simulink model "Feedforward_completo"  (R2021b)
settings: Solver=VariableStepAuto  StartTime=0.0  StopTime=10.0  RelTol=1e-3
PreLoadFcn:
  | Fs = 44100;
  | f_tono = 500;
  | L = 32;
InitFcn:
  | Fs = 44100;
  | f_tono = 500;
  | L = 32;
undefined symbols (not defined in the file or in its folder): SzEstimado
settings Model: Creator=Vale Oieni  LastModifiedBy=ValeOieni

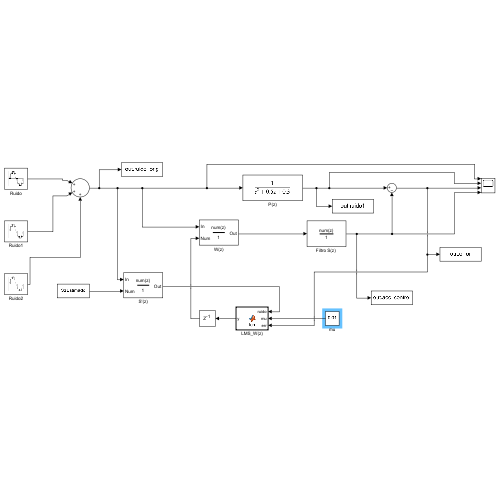
[thumbnail: Simulink's stored preview of the top-level diagram]
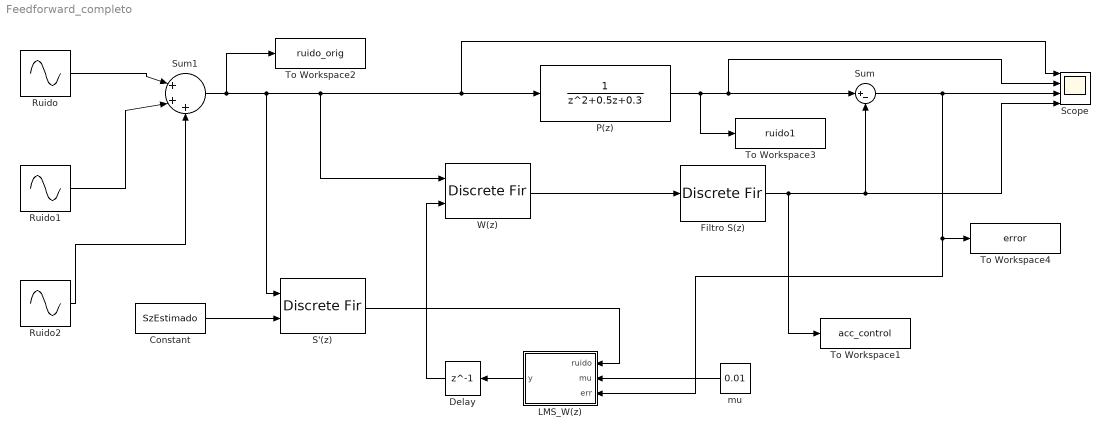
== system Feedforward_completo ==
  Constant : Constant  Value=SzEstimado  SampleTime=1/Fs
  Delay : Delay  DelayLength=1  InitialCondition=0  SampleTime=1/Fs
  "Filtro S(z) " : DiscreteFir  Coefficients=[0 0 -.5 .5 -.3 .2 -.1 .5 -.5]  InputProcessing=Columns as channels (frame based)  SampleTime=1/Fs
  LMS_W(z) : MATLAB Function  TreatAsAtomicUnit=on
  P(z) : DiscreteTransferFcn  Denominator="[1 0.5  0.3]"
  Ruido : Sin  Frequency=f_tono*(2*pi)  SampleTime=1/Fs
  Ruido1 : Sin  Frequency=2*f_tono*(2*pi)  SampleTime=1/Fs
  Ruido2 : Sin  Amplitude=2  Frequency=0.3*f_tono*(2*pi)  SampleTime=1/Fs
  S'(z) : DiscreteFir  CoefSource=Input port  InputProcessing=Columns as channels (frame based)  SampleTime=1/Fs
      settings: InputPortMap=u0,u1
  Scope : Scope  NumInputPorts=4
  Sum : Sum  Inputs=|+-
  Sum1 : Sum  Inputs=|+++
  To Workspace1 : ToWorkspace  VariableName=acc_control  SampleTime=-1
      settings: Save2DSignal=2-D array (concatenate along first dimension)
  To Workspace2 : ToWorkspace  VariableName=ruido_orig  SampleTime=-1
      settings: Save2DSignal=2-D array (concatenate along first dimension)
  To Workspace3 : ToWorkspace  VariableName=ruido1  SampleTime=-1
      settings: Save2DSignal=2-D array (concatenate along first dimension)
  To Workspace4 : ToWorkspace  VariableName=error  SampleTime=-1
      settings: Save2DSignal=2-D array (concatenate along first dimension)
  W(z) : DiscreteFir  CoefSource=Input port  SampleTime=1/Fs
      settings: InputPortMap=u0,u1
  mu : Constant  Value=0.01  SampleTime=1/Fs
  wires:
  P(z)/1 -> To Workspace3/1, Scope/2, Sum/1
  Sum/1 -> Scope/3, To Workspace4/1, LMS_W(z)/3(err)
  "Filtro S(z) "/1 -> To Workspace1/1, Scope/4, Sum/2
  Ruido/1 -> Sum1/1
  Ruido1/1 -> Sum1/2
  Ruido2/1 -> Sum1/3
  Sum1/1 -> To Workspace2/1, S'(z)/1, Scope/1, P(z)/1, W(z)/1
  W(z)/1 -> "Filtro S(z) "/1
  Constant/1 -> S'(z)/2
  S'(z)/1 -> LMS_W(z)/1(ruido)
  mu/1 -> LMS_W(z)/2(mu)
  LMS_W(z)/1(y) -> Delay/1
  Delay/1 -> W(z)/2

== matlab function Feedforward_completo/LMS_W(z) ==
  data: ruido input; mu input; y output; err input
function y = fcn(ruido, mu, err)
    L = 32;
    %Pesos w_n
    persistent w_n
    if isempty(w_n)
        w_n = zeros(1, L); % inicializa w en cero, largo L
    end
    %Vector de ruido
    persistent x
    if isempty(x)
        x = zeros(1, L); % inicializa x en cero, largo L
    end
    %Vaciado de x
    x(2:L) = x(1:L-1);
    x(1) = ruido;
    %Actualizacion
    xvar = x;
    w = w_n;
    w = w + mu*err*xvar;   
    w_n = w;
    %Asignación a la salida
    y = w;
end
